simulink model "PDGF"  (R2021b)
settings: Solver=VariableStepAuto  StartTime=0.0  StopTime=15  RelTol=1e-3
values from neighbouring files (symbols this model uses):
  dq_i = zeros(6,1)    [PDGC_main.m]
  F_v = zeros(6,6)    [PDGC_main.m]
  K_d = 20.*eye(6,6)    [PDGC_main.m]
  K_p = 100.*eye(6,6)    [PDGC_main.m]
  max_torques = 0.75*[97.6 186.4 89.4 24.2 20.1 21.3]'    [PDGC_main.m]
  min_torques = -0.75*[97.6 186.4 89.4 24.2 20.1 21.3]'    [PDGC_main.m]
  q_i = zeros(6,1)    [PDGC_main.m]
settings Model: Creator=ASUS  LastModifiedBy=ASUS

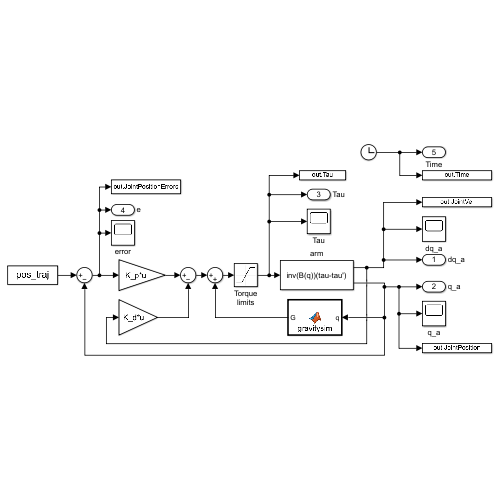
[thumbnail: Simulink's stored preview of the top-level diagram]
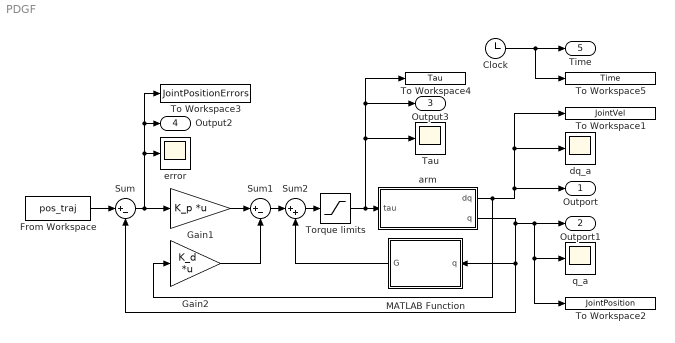
== system PDGF ==
  Clock : Clock
  From Workspace : FromWorkspace  VariableName=pos_traj  OutputAfterFinalValue=Holding final value
  Gain1 : Gain  Gain=K_p  Multiplication=Matrix(K*u)
  Gain2 : Gain  Gain=K_d  Multiplication=Matrix(K*u)
  MATLAB Function : MATLAB Function  TreatAsAtomicUnit=on
  Sum : Sum  Inputs=|+-
  Sum1 : Sum  Inputs=|+-
  Sum2 : Sum  Inputs=|++
  Tau : Scope
  To Workspace1 : ToWorkspace  VariableName=JointVel  SaveFormat=Timeseries  SampleTime=-1
  To Workspace2 : ToWorkspace  VariableName=JointPosition  SaveFormat=Timeseries  SampleTime=-1
  To Workspace3 : ToWorkspace  VariableName=JointPositionErrors  SaveFormat=Timeseries  SampleTime=-1
  To Workspace4 : ToWorkspace  VariableName=Tau  SaveFormat=Timeseries  SampleTime=-1
  To Workspace5 : ToWorkspace  VariableName=Time  SaveFormat=Timeseries  SampleTime=-1
  Torque limits : Saturate  UpperLimit=max_torques  LowerLimit=min_torques
  arm : Subsystem
      mask Display: disp('inv(B(q))(tau-tau'')')
  dq_a : Scope
  error : Scope
  q_a : Scope
  Outport : Outport  SignalName=dq_a
  Outport1 : Outport  Port=2  SignalName=q_a
  Output3 : Outport  Port=3  SignalName=Tau
  Output2 : Outport  Port=4  SignalName=e
  Time : Outport  Port=5
  wires:
  Sum1/1 -> Sum2/1
  MATLAB Function/1(G) -> Sum2/2
  Gain1/1 -> Sum1/1
  Gain2/1 -> Sum1/2
  From Workspace/1 -> Sum/1
  Sum2/1 -> Torque limits/1
  Torque limits/1 -> Tau/1, To Workspace4/1, Output3/1, arm/1(tau)
  Sum/1 -> To Workspace3/1, Output2/1, error/1, Gain1/1
  Clock/1 -> To Workspace5/1, Time/1
  arm/1(dq) -> To Workspace1/1, dq_a/1, Outport/1, Gain2/1
  arm/2("q ") -> Outport1/1, To Workspace2/1, q_a/1, Sum/2, MATLAB Function/1(q)

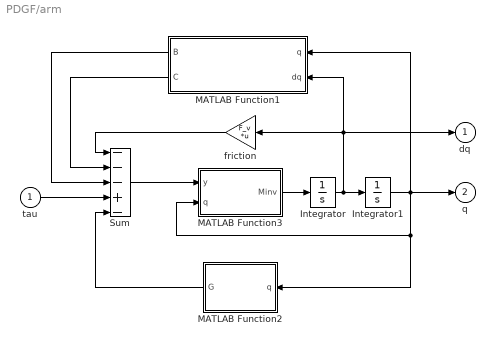
== system PDGF/arm ==
  tau : Inport
  Integrator : Integrator  InitialCondition=dq_i  ZeroCross=off
  Integrator1 : Integrator  InitialCondition=q_i  ZeroCross=off
  MATLAB Function1 : MATLAB Function  TreatAsAtomicUnit=on
  MATLAB Function2 : MATLAB Function  TreatAsAtomicUnit=on
  MATLAB Function3 : MATLAB Function  TreatAsAtomicUnit=on
  Sum : Sum  Inputs=---+-  InputSameDT=on  SaturateOnIntegerOverflow=on  OutDataTypeStr=Inherit: Same as first input
  friction : Gain  Gain=F_v  Multiplication=Matrix(K*u)  SaturateOnIntegerOverflow=on  OutDataTypeStr=Inherit: Same as input  ParamDataTypeStr=Inherit: Same as input
      mask Display: disp('F_v')
  dq : Outport  InitialOutput=0
  "q " : Outport  Port=2  InitialOutput=0
  wires:
  Integrator1/1 -> MATLAB Function1/1(q), MATLAB Function2/1(q), MATLAB Function3/2(q), "q "/1
  MATLAB Function3/1(Minv) -> Integrator/1
  Integrator/1 -> Integrator1/1, dq/1, MATLAB Function1/2(dq), friction/1
  Sum/1 -> MATLAB Function3/1(y)
  friction/1 -> Sum/1
  MATLAB Function2/1(G) -> Sum/5
  tau/1 -> Sum/4
  MATLAB Function1/1(B) -> Sum/3
  MATLAB Function1/2(C) -> Sum/2

== matlab function PDGF/arm/MATLAB Function1 ==
  data: q input; B output; dq input; C output
function [B,C] = corioliscentrifugalsim(q, dq)
[B,C] = corioliscentrifugal(q, dq);
end

== matlab function PDGF/arm/MATLAB Function2 ==
  data: q input; G output
function G = gravitysim(q)
G = gravity(q);
end

== matlab function PDGF/arm/MATLAB Function3 ==
  data: y input; q input; Minv output
function Minv = inertiainvsim(y, q)
M = inertia(q);
% M=M(1:3,1:3);
Minv = inv(M)*y;

end

== matlab function PDGF/MATLAB Function ==
  data: q input; G output
function G = gravitysim(q)
G = gravity(q);
end
